simulink model "SCT_mdl"  (R2017a)
settings: Solver=VariableStepAuto  StartTime=0.0  StopTime=10.0  RelTol=1e-3
values from neighbouring files (symbols this model uses):
  beta_14 = 0.23    [HuiL_HVAC_mdl_all_sim.m]
  beta_21 = 0.3    [HuiL_HVAC_mdl_all_sim.m]
  beta_25 = 0.3    [HuiL_HVAC_mdl_all_sim.m]
  beta_31 = 0.5    [HuiL_HVAC_mdl_all_sim.m]
  beta_34 = 0.2    [HuiL_HVAC_mdl_all_sim.m]
  beta_42 = 0.3    [HuiL_HVAC_mdl_all_sim.m]
  beta_43 = 0.8    [HuiL_HVAC_mdl_all_sim.m]
  beta_45 = 0.0    (= 0)    [HuiL_HVAC_mdl_all_sim.m]
  beta_46 = 0.55    [HuiL_HVAC_mdl_all_sim.m]
  beta_54 = 0.3    [HuiL_HVAC_mdl_all_sim.m]
  eta_0 = zeros(6,1)    [HuiL_HVAC_mdl_all_sim.m]
  gamma_11 = 0.8    [HuiL_HVAC_mdl_all_sim.m]
  gamma_22 = 0.75    [HuiL_HVAC_mdl_all_sim.m]
  gamma_32 = 1.6    [HuiL_HVAC_mdl_all_sim.m]
  gamma_33 = 0.75    [HuiL_HVAC_mdl_all_sim.m]
  gamma_35 = 1    [HuiL_HVAC_mdl_all_sim.m]
  gamma_36 = 1    [HuiL_HVAC_mdl_all_sim.m]
  gamma_57 = 2    [HuiL_HVAC_mdl_all_sim.m]
  gamma_64 = 20    [HuiL_HVAC_mdl_all_sim.m]
  gamma_68 = 5    [HuiL_HVAC_mdl_all_sim.m]
  tau = 0.1*[     1 ... (first row only)    [HuiL_HVAC_mdl_all_sim.m]
  theta = zeros(19,1)    [HuiL_HVAC_mdl_all_sim.m]
  zeta_var = 0    [HuiL_HVAC_mdl_all_sim.m]
settings Model: Creator=thisi  LastModifiedBy=thisi

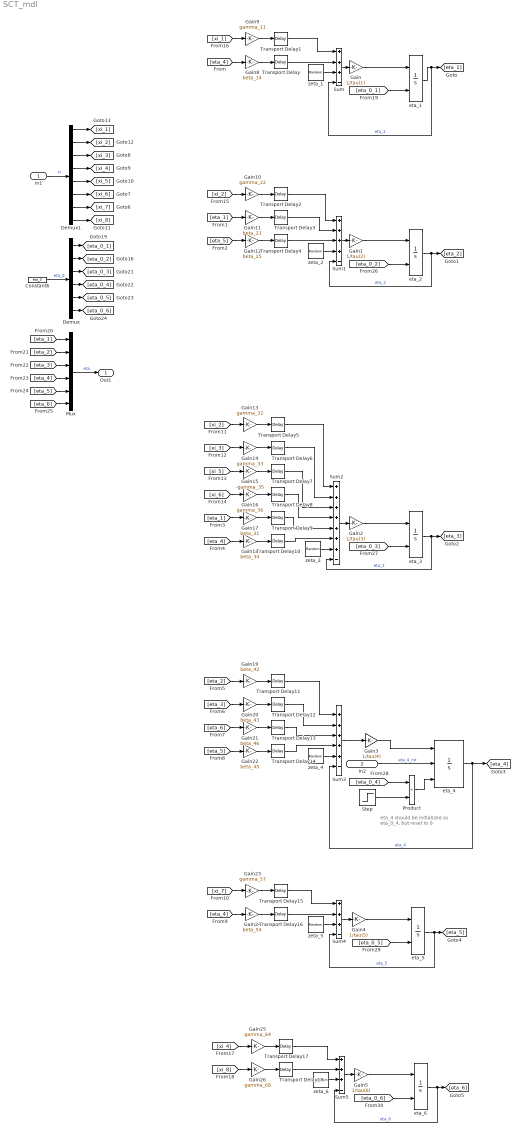
== system SCT_mdl ==
  note: eta_4 should be initialized
      | as eta_0_4, but reset to 0
  In1 : Inport
  In2 : Inport  Port=2
  Constant6 : Constant  Value=eta_0
  Demux : Demux  Outputs=6
  Demux1 : Demux  Outputs=8
  Gain : Gain  Gain=1/tau(1)
      settings: AttributesFormatString=%<Gain>
  Gain1 : Gain  Gain=1/tau(2)
      settings: AttributesFormatString=%<Gain>
  Gain10 : Gain  Gain=gamma_22
      settings: AttributesFormatString=%<Gain>
  Gain11 : Gain  Gain=beta_21
      settings: AttributesFormatString=%<Gain>
  Gain12 : Gain  Gain=beta_25
      settings: AttributesFormatString=%<Gain>
  Gain13 : Gain  Gain=gamma_32
      settings: AttributesFormatString=%<Gain>
  Gain14 : Gain  Gain=gamma_33
      settings: AttributesFormatString=%<Gain>
  Gain15 : Gain  Gain=-gamma_35
      settings: AttributesFormatString=%<Gain>
  Gain16 : Gain  Gain=gamma_36
      settings: AttributesFormatString=%<Gain>
  Gain17 : Gain  Gain=beta_31
      settings: AttributesFormatString=%<Gain>
  Gain18 : Gain  Gain=beta_34
      settings: AttributesFormatString=%<Gain>
  Gain19 : Gain  Gain=beta_42
      settings: AttributesFormatString=%<Gain>
  Gain2 : Gain  Gain=1/tau(3)
      settings: AttributesFormatString=%<Gain>
  Gain20 : Gain  Gain=beta_43
      settings: AttributesFormatString=%<Gain>
  Gain21 : Gain  Gain=beta_46
      settings: AttributesFormatString=%<Gain>
  Gain22 : Gain  Gain=beta_45
      settings: AttributesFormatString=%<Gain>
  Gain23 : Gain  Gain=gamma_57
      settings: AttributesFormatString=%<Gain>
  Gain24 : Gain  Gain=beta_54
      settings: AttributesFormatString=%<Gain>
  Gain25 : Gain  Gain=gamma_64
      settings: AttributesFormatString=%<Gain>
  Gain26 : Gain  Gain=gamma_68
      settings: AttributesFormatString=%<Gain>
  Gain3 : Gain  Gain=1/tau(4)
      settings: AttributesFormatString=%<Gain>
  Gain4 : Gain  Gain=1/tau(5)
      settings: AttributesFormatString=%<Gain>
  Gain5 : Gain  Gain=1/tau(6)
      settings: AttributesFormatString=%<Gain>
  Gain8 : Gain  Gain=beta_14
      settings: AttributesFormatString=%<Gain>
  Gain9 : Gain  Gain=gamma_11
      settings: AttributesFormatString=%<Gain>
  Mux : Mux  Inputs=6
  Product : Product
  Step : Step  Time=0.1  Before=1  After=0  SampleTime=0
  Sum : Sum  Inputs=+++-
  Sum1 : Sum  Inputs=++++-
  Sum2 : Sum  Inputs=+++++++-
  Sum3 : Sum  Inputs=+++++-
  Sum4 : Sum  Inputs=+++-
  Sum5 : Sum  Inputs=+++-
  Transport Delay : TransportDelay  DelayTime=theta(16)
      settings: AttributesFormatString=%<DelayTime>
  Transport Delay1 : TransportDelay  DelayTime=theta(1)
      settings: AttributesFormatString=%<DelayTime>
  Transport Delay10 : TransportDelay  DelayTime=theta(13)
      settings: AttributesFormatString=%<DelayTime>
  Transport Delay11 : TransportDelay  DelayTime=theta(6)
      settings: AttributesFormatString=%<DelayTime>
  Transport Delay12 : TransportDelay  DelayTime=theta(8)
      settings: AttributesFormatString=%<DelayTime>
  Transport Delay13 : TransportDelay  DelayTime=theta(17)
      settings: AttributesFormatString=%<DelayTime>
  Transport Delay14 : TransportDelay  DelayTime=theta(19)
      settings: AttributesFormatString=%<DelayTime>
  Transport Delay15 : TransportDelay  DelayTime=theta(15)
      settings: AttributesFormatString=%<DelayTime>
  Transport Delay16 : TransportDelay  DelayTime=theta(12)
      settings: AttributesFormatString=%<DelayTime>
  Transport Delay17 : TransportDelay  DelayTime=theta(11)
      settings: AttributesFormatString=%<DelayTime>
  Transport Delay18 : TransportDelay  DelayTime=theta(18)
      settings: AttributesFormatString=%<DelayTime>
  Transport Delay2 : TransportDelay  DelayTime=theta(4)
      settings: AttributesFormatString=%<DelayTime>
  Transport Delay3 : TransportDelay  DelayTime=theta(2)
      settings: AttributesFormatString=%<DelayTime>
  Transport Delay4 : TransportDelay  DelayTime=theta(14)
      settings: AttributesFormatString=%<DelayTime>
  Transport Delay5 : TransportDelay  DelayTime=theta(5)
      settings: AttributesFormatString=%<DelayTime>
  Transport Delay6 : TransportDelay  DelayTime=theta(7)
      settings: AttributesFormatString=%<DelayTime>
  Transport Delay7 : TransportDelay  DelayTime=theta(9)
      settings: AttributesFormatString=%<DelayTime>
  Transport Delay8 : TransportDelay  DelayTime=theta(10)
      settings: AttributesFormatString=%<DelayTime>
  Transport Delay9 : TransportDelay  DelayTime=theta(3)
      settings: AttributesFormatString=%<DelayTime>
  eta_1 : Integrator  InitialConditionSource=external  InitialCondition=eta_0(1)  LimitOutput=on  UpperSaturationLimit=100  LowerSaturationLimit=0  ContinuousStateAttributes='eta_1'
  eta_2 : Integrator  InitialConditionSource=external  InitialCondition=eta_0(1)  LimitOutput=on  UpperSaturationLimit=100  LowerSaturationLimit=0  ContinuousStateAttributes='eta_2'
  eta_3 : Integrator  InitialConditionSource=external  InitialCondition=eta_0(1)  LimitOutput=on  UpperSaturationLimit=100  LowerSaturationLimit=0  ContinuousStateAttributes='eta_3'
  eta_4 : Integrator  ExternalReset=rising  InitialConditionSource=external  InitialCondition=eta_0(1)  LimitOutput=on  UpperSaturationLimit=100  LowerSaturationLimit=0  ContinuousStateAttributes='eta_4'
  eta_5 : Integrator  InitialConditionSource=external  InitialCondition=eta_0(1)  LimitOutput=on  UpperSaturationLimit=100  LowerSaturationLimit=0  ContinuousStateAttributes='eta_5'
  eta_6 : Integrator  InitialConditionSource=external  InitialCondition=eta_0(1)  LimitOutput=on  UpperSaturationLimit=100  LowerSaturationLimit=0  ContinuousStateAttributes='eta_6'
  zeta_{1..6} (6 alike) : RandomNumber  Variance=zeta_var  SampleTime=0.1
  Out1 : Outport
  wires:
  [eta_0_6] -> eta_6/2
  Demux1/4 -> [xi_4]
  Demux1/8 -> [xi_8]
  Gain9/1 -> Transport Delay1/1
  [eta_3] -> Mux/3
  Gain5/1 -> eta_6/1
  Demux/4 -> [eta_0_4]
  [eta_2] -> Gain19/1
  [eta_2] -> Mux/2
  Demux1/5 -> [xi_5]
  [eta_6] -> Mux/6
  Demux1/7 -> [xi_7]
  Transport Delay1/1 -> Sum/1
  Gain20/1 -> Transport Delay12/1
  Gain15/1 -> Transport Delay7/1
  [xi_4] -> Gain25/1
  [eta_0_2] -> eta_2/2
  Demux/3 -> [eta_0_3]
  Constant6/1 -> Demux/1  "eta_0"
  [eta_5] -> Mux/5
  Gain12/1 -> Transport Delay4/1
  [eta_4] -> Gain18/1
  Transport Delay10/1 -> Sum2/6
  Transport Delay11/1 -> Sum3/1
  Gain8/1 -> Transport Delay/1
  Gain19/1 -> Transport Delay11/1
  zeta_1/1 -> Sum/3
  Transport Delay13/1 -> Sum3/3
  [eta_1] -> Mux/1
  Gain2/1 -> eta_3/1
  Transport Delay15/1 -> Sum4/1
  eta_6/1 -> [eta_6], Sum5/4  "eta_6"
  Transport Delay4/1 -> Sum1/3
  Transport Delay3/1 -> Sum1/2
  [eta_0_4] -> Product/1
  Transport Delay9/1 -> Sum2/5
  Demux1/6 -> [xi_6]
  Gain11/1 -> Transport Delay3/1
  zeta_4/1 -> Sum3/5
  Demux/1 -> [eta_0_1]
  Demux1/3 -> [xi_3]
  [eta_4] -> Mux/4
  [eta_1] -> Gain17/1
  Demux1/2 -> [xi_2]
  Transport Delay5/1 -> Sum2/1
  [eta_0_3] -> eta_3/2
  [eta_0_5] -> eta_5/2
  [eta_0_1] -> eta_1/2
  Gain3/1 -> eta_4/1
  Demux/5 -> [eta_0_5]
  zeta_3/1 -> Sum2/7
  Gain24/1 -> Transport Delay16/1
  [eta_4] -> Gain8/1
  Transport Delay18/1 -> Sum5/2
  Sum1/1 -> Gain1/1
  zeta_5/1 -> Sum4/3
  Sum/1 -> Gain/1
  Gain18/1 -> Transport Delay10/1
  Transport Delay6/1 -> Sum2/2
  Gain1/1 -> eta_2/1
  Sum3/1 -> Gain3/1
  Sum2/1 -> Gain2/1
  zeta_2/1 -> Sum1/4
  Transport Delay14/1 -> Sum3/4
  eta_1/1 -> [eta_1], Sum/4  "eta_1"
  Gain16/1 -> Transport Delay8/1
  Gain14/1 -> Transport Delay6/1
  Transport Delay12/1 -> Sum3/2
  Transport Delay7/1 -> Sum2/3
  [eta_3] -> Gain20/1
  [xi_5] -> Gain15/1
  Sum4/1 -> Gain4/1
  [eta_4] -> Gain24/1
  Gain25/1 -> Transport Delay17/1
  [eta_1] -> Gain11/1
  Transport Delay16/1 -> Sum4/2
  Transport Delay17/1 -> Sum5/1
  [xi_7] -> Gain23/1
  Gain21/1 -> Transport Delay13/1
  [xi_1] -> Gain9/1
  Transport Delay2/1 -> Sum1/1
  Gain26/1 -> Transport Delay18/1
  [xi_6] -> Gain16/1
  Transport Delay/1 -> Sum/2
  Demux1/1 -> [xi_1]
  Demux/2 -> [eta_0_2]
  Gain/1 -> eta_1/1
  eta_4/1 -> Sum3/6, [eta_4]  "eta_4"
  Gain4/1 -> eta_5/1
  Mux/1 -> Out1/1  "eta"
  [xi_2] -> Gain10/1
  [eta_6] -> Gain21/1
  Gain23/1 -> Transport Delay15/1
  eta_2/1 -> [eta_2], Sum1/5  "eta_2"
  Transport Delay8/1 -> Sum2/4
  [xi_8] -> Gain26/1
  [xi_2] -> Gain13/1
  eta_3/1 -> [eta_3], Sum2/8  "eta_3"
  [eta_5] -> Gain12/1
  In1/1 -> Demux1/1  "xi"
  Gain13/1 -> Transport Delay5/1
  [eta_5] -> Gain22/1
  Gain22/1 -> Transport Delay14/1
  zeta_6/1 -> Sum5/3
  Demux/6 -> [eta_0_6]
  eta_5/1 -> [eta_5], Sum4/4  "eta_5"
  In2/1 -> eta_4/2  "eta_4_rst"
  Gain17/1 -> Transport Delay9/1
  Sum5/1 -> Gain5/1
  [xi_3] -> Gain14/1
  Gain10/1 -> Transport Delay2/1
  Step/1 -> Product/2
  Product/1 -> eta_4/3
